simulink model "ms_inter2"  (Simulink 7.3)
settings: Solver=VariableStepDiscrete  StartTime=0.0  StopTime=10.0  MaxStep=0.1  RelTol=1e-3
settings Model: Creator=sn00632  LastModifiedBy=sn00632

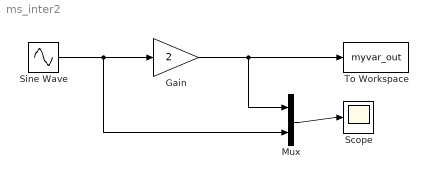
== system ms_inter2 ==
  Gain : Gain  Gain=2  ParameterDataType=fixdt(1, 16)  ParameterScaling=2^0  OutDataType=fixdt(1, 16)  OutScaling=2^0
  Mux : Mux  Inputs=2
  Scope : Scope
  Sine Wave : Sin  Amplitude=1  Bias=0  Frequency=1  Phase=0  Samples=10  SampleTime=0  Offset=0
  To Workspace : ToWorkspace  VariableName=myvar_out  SampleTime=-1  SaveFormat=Structure
  wires:
  Sine Wave/1 -> Gain/1, Mux/2
  Gain/1 -> Mux/1, To Workspace/1
  Mux/1 -> Scope/1
